simulink model "Surge_velocity_control"  (R2023a)
settings: Solver=VariableStepAuto  StartTime=0.0  StopTime=10.0  RelTol=1e-3
settings Model: Creator=Ask for  LastModifiedBy=Ask for

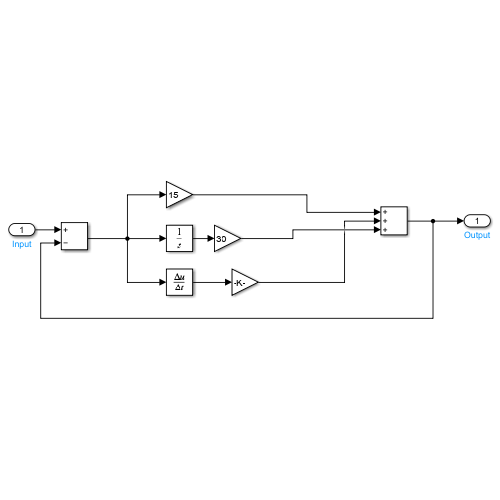
[thumbnail: Simulink's stored preview of the top-level diagram]
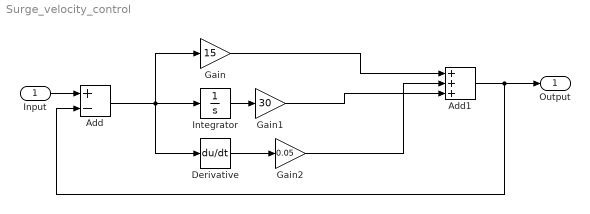
== system Surge_velocity_control ==
  Input : Inport
  Add : Sum  Inputs=+-
  Add1 : Sum  Inputs=+++
  Derivative : Derivative  CoefficientInTFapproximation=0
  Gain : Gain  Gain=15
  Gain1 : Gain  Gain=30
  Gain2 : Gain  Gain=0.05
  Integrator : Integrator
  Output : Outport
  wires:
  Integrator/1 -> Gain1/1
  Derivative/1 -> Gain2/1
  Gain/1 -> Add1/1
  Gain1/1 -> Add1/3
  Gain2/1 -> Add1/2
  Add/1 -> Gain/1, Integrator/1, Derivative/1
  Add1/1 -> Output/1, Add/2
  Input/1 -> Add/1
